simulink model "UltrasonicMux_Module"  (R2021b)
settings: Solver=FixedStepAuto  StartTime=0.0  StopTime=inf  FixedStep=0.01  RelTol=1e-3  EnableMultiTasking=on
libraries: arduinosensorlib x3
settings Model: ExtModeTrigDuration=2  Creator=user  LastModifiedBy=user
settings OptimizationCC: EnhancedBackFolding=on  PassReuseOutputArgsAs=Individual arguments  ZeroExternalMemoryAtStartup=off  ZeroInternalMemoryAtStartup=off  MaxStackSize=64  OptimizeBlockOrder=speed  DifferentSizesBufferReuse=on  OptimizationCustomize=off  EfficientTunableParamExpr=on
settings DebuggingCC: MultiTaskDSMMsg=none  ParameterTunabilityLossMsg=error
settings HardwareCC: ProdBitPerInt=16  ProdBitPerPointer=16  ProdBitPerSizeT=16  ProdBitPerPtrDiffT=16  ProdLargestAtomicFloat=None  ProdWordSize=8  ProdHWDeviceType=Atmel->AVR
settings SFSimCC: MATLABDynamicMemAlloc=off
settings RTWCC: Description=Embedded Coder  SystemTargetFile=ert.tlc  HardwareBoard=Arduino Mega 2560  TemplateMakefile=ert_default_tmf  Toolchain=Arduino AVR  BuildConfiguration=Faster Runs
settings CodeAppCC: ForceParamTrailComments=on  IgnoreCustomStorageClasses=off  OperatorAnnotations=on  SimulinkDataObjDesc=on  SFDataObjDesc=on  InsertBlockDesc=on
settings ERTTargetCC: SupportContinuousTime=on  SupportVariableSizeSignals=on  ExtModeTransport=3  ExtModeStaticAlloc=on  ExtModeStaticAllocSize=2048  ExtModeMexFile=ext_xcp  ExtModeIntrfLevel=Level2 - Open

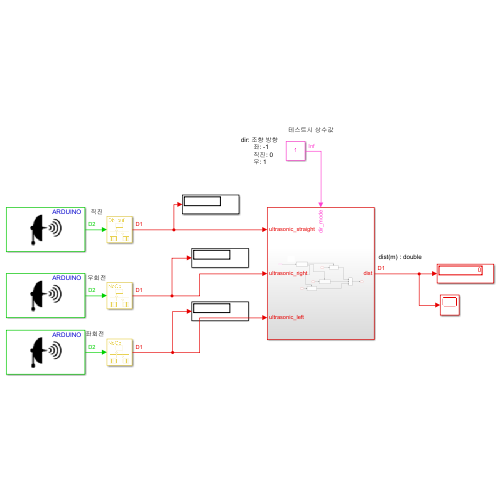
[thumbnail: Simulink's stored preview of the top-level diagram]
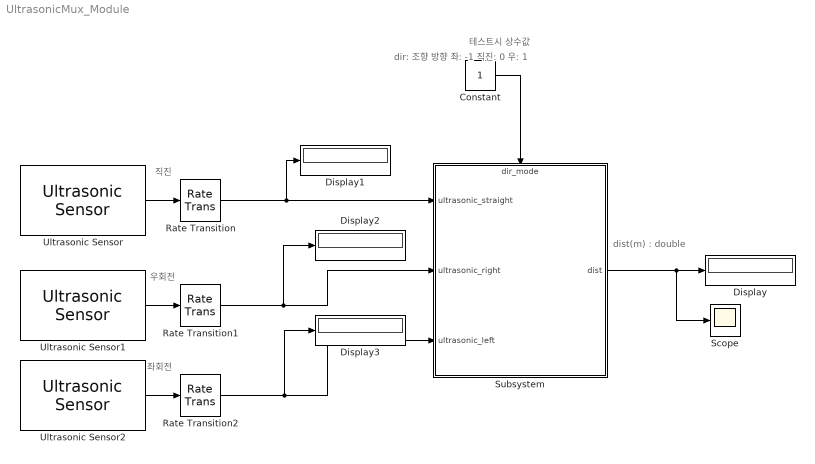
== system UltrasonicMux_Module ==
  note: dist(m) : double
  note: 테스트시 상수값
  note: dir: 조향 방향
      |  	좌: -1
      |  	직진: 0
      |  	우: 1
  note: 우회전
  note: 좌회전
  note: 직진
  Constant : Constant
  Display{,1..3} (4 alike) : Display
  Rate Transition : RateTransition  Deterministic=off  OutPortSampleTime=0.01
  Rate Transition1 : RateTransition  Deterministic=off  OutPortSampleTime=0.01
  Rate Transition2 : RateTransition  Deterministic=off  OutPortSampleTime=0.01
  Scope : Scope
  Subsystem : Subsystem
      settings: PortSchema="{\"entries\":[{\"content\":{\"sides\":[{\"content\":{\"connectorIds\":[\"In1\",\"In2\",\"In3\"]},\"type\":\"ConnectorPlacement.EquallySpacedRectSide\",\"uuid\":\"5f4ad8f0-04c3-4479-9dfd-33641402f242\"},{\"content\":{\"connectorIds\":[\"Out1\"],\"side\":\"RIGHT\"},\"type\":\"ConnectorPlacement.EquallySpacedRectSide\",\"uuid\":\"c4451af6-64c8-402e-8ffe-feeed5b209e6\"},{\"content\":{\"connectorIds\":[\"In4\"],\"side\":\"TOP\"},\"type\":\"ConnectorPlacement.EquallySpacedRectSide\",\"uuid\":\"4be8f8c7-8102-4379-8072-e8a8027f489d\"}]},\"type\":\"ConnectorPlacement.EquallySpacedConnector\",\"uuid\":\"2bd08bb9-e7f4-4004-b808-4b0f9daf5a96\"}],\"packageUris\":[\"http://schema.mathworks.com/mf0/Connector/R2020b\"],\"version\":\"1.0\"}"
  Ultrasonic Sensor : arduinosensorlib/Ultrasonic Sensor  NumSignalPins=2  TrigPin=50  EchoPin=51  SignalPin=3  SampleTime_=0.1  blockPlatform=ARDUINO
      settings: SourceProductBaseCode=ARDUINO
  Ultrasonic Sensor1 : arduinosensorlib/Ultrasonic Sensor  NumSignalPins=2  TrigPin=48  EchoPin=49  SignalPin=3  SampleTime_=0.1  blockPlatform=ARDUINO
      settings: SourceProductBaseCode=ARDUINO
  Ultrasonic Sensor2 : arduinosensorlib/Ultrasonic Sensor  NumSignalPins=2  TrigPin=46  EchoPin=47  SignalPin=3  SampleTime_=0.1  blockPlatform=ARDUINO
      settings: SourceProductBaseCode=ARDUINO
  wires:
  Ultrasonic Sensor/1 -> Rate Transition/1
  Ultrasonic Sensor1/1 -> Rate Transition1/1
  Ultrasonic Sensor2/1 -> Rate Transition2/1
  Rate Transition/1 -> Display1/1, Subsystem/1(ultrasonic_straight)
  Rate Transition1/1 -> Display2/1, Subsystem/2(ultrasonic_right)
  Rate Transition2/1 -> Display3/1, Subsystem/3(ultrasonic_left)
  Constant/1 -> Subsystem/4(dir_mode)
  Subsystem/1(dist) -> Scope/1, Display/1

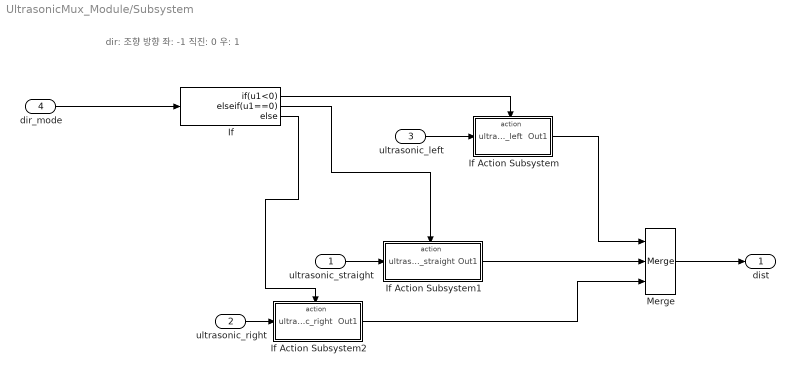
== system UltrasonicMux_Module/Subsystem ==
  note: dir: 조향 방향
      |  	좌: -1
      |  	직진: 0
      |  	우: 1
  ultrasonic_straight : Inport
  ultrasonic_right : Inport  Port=2
  ultrasonic_left : Inport  Port=3
  dir_mode : Inport  Port=4
  If : If  IfExpression=u1<0  ElseIfExpressions=u1==0
  If Action Subsystem : Subsystem  TreatAsAtomicUnit=on
  If Action Subsystem1 : Subsystem  TreatAsAtomicUnit=on
  If Action Subsystem2 : Subsystem  TreatAsAtomicUnit=on
  Merge : Merge  Inputs=3
  dist : Outport
  wires:
  dir_mode/1 -> If/1
  If/1 -> If Action Subsystem/Action
  ultrasonic_left/1 -> If Action Subsystem/1(ultrasonic_left)
  If/2 -> If Action Subsystem1/Action
  ultrasonic_straight/1 -> If Action Subsystem1/1(ultrasonic_straight)
  If/3 -> If Action Subsystem2/Action
  ultrasonic_right/1 -> If Action Subsystem2/1(ultrasonic_right)
  If Action Subsystem1/1(Out1) -> Merge/2
  If Action Subsystem2/1(Out1) -> Merge/3
  If Action Subsystem/1(Out1) -> Merge/1
  Merge/1 -> dist/1

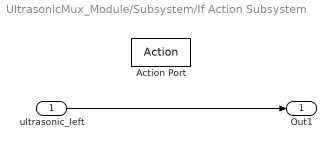
== system UltrasonicMux_Module/Subsystem/If Action Subsystem ==
  ultrasonic_left : Inport
  Action Port : ActionPort  ActionPortLabel=if(u1<0)
  Out1 : Outport
  wires:
  ultrasonic_left/1 -> Out1/1

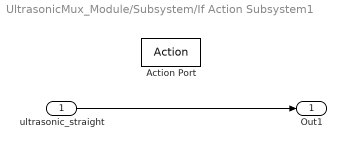
== system UltrasonicMux_Module/Subsystem/If Action Subsystem1 ==
  ultrasonic_straight : Inport
  Action Port : ActionPort  ActionPortLabel=elseif(u1==0)
  Out1 : Outport
  wires:
  ultrasonic_straight/1 -> Out1/1

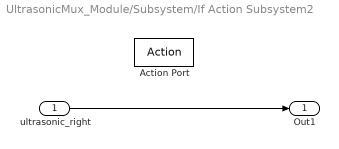
== system UltrasonicMux_Module/Subsystem/If Action Subsystem2 ==
  ultrasonic_right : Inport
  Action Port : ActionPort  ActionPortLabel=else
  Out1 : Outport
  wires:
  ultrasonic_right/1 -> Out1/1
